simulink model "gm_uz_pmsm_model_9ph"  (R2021b)
settings: Solver=FixedStepAuto  StartTime=0.0  StopTime=0.8  RelTol=1e-3
PreLoadFcn:
  | uz_pmsm_model_9ph_init_parameter
undefined symbols (not defined in the file or in its folder): a, b, c, friction_coefficient, inertia, k_i_d, k_i_q, k_p_d, k_p_q, Kpd, L_d, L_o1, L_o2, L_q, L_x1, L_x2, L_y1, L_y2, L_zero, polepair, psi_pm, R_1, static_friction_torque, Tnd
libraries: hdlmdlgenlib x190, hdlsllib x90, dspsigops x17, simulink x3, slpidlib x2, spsAlphaBetaZerotodq0Lib x1, pid_lib x1, spsdq0toAlphaBetaZeroLib x1
(part 5 of 6)

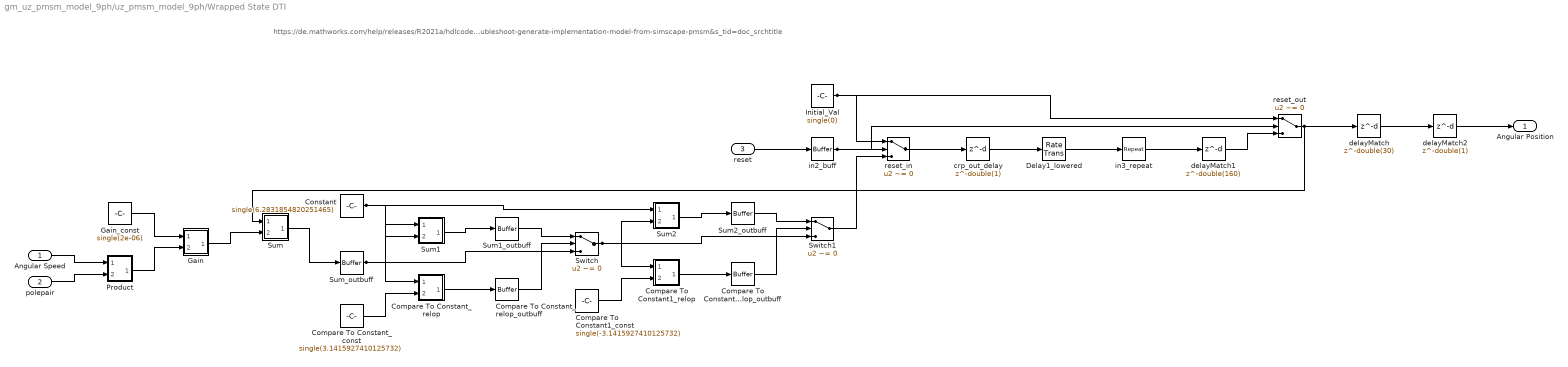
== system gm_uz_pmsm_model_9ph/uz_pmsm_model_9ph/Wrapped State DTI ==
  note: https://de.mathworks.com/help/releases/R2021a/hdlcoder/ug/troubleshoot-generate-implementation-model-from-simscape-pmsm.html?searchHighlight=troubleshoot-generate-implementation-model-from-simscape-pmsm&s_tid=doc_srchtitle
  Angular Speed : Inport  OutDataTypeStr=single  PortDimensions=1  SampleTime=1e-08
  polepair : Inport  Port=2  OutDataTypeStr=single  PortDimensions=1  SampleTime=1e-08
  reset : Inport  Port=3  OutDataTypeStr=boolean  PortDimensions=1  SampleTime=1e-08
  Compare To Constant1_const : Constant  Value=single(-3.1415927410125732)  OutDataTypeStr=single  SampleTime=1e-08
  Compare To Constant1_relop : Subsystem
      mask Display: disp('NFP\nrelop');
  Compare To Constant1_relop_outbuff : hdlmdlgenlib/Buffer
      settings: SourceProductBaseCode=SL
  Compare To Constant_const : Constant  Value=single(3.1415927410125732)  OutDataTypeStr=single  SampleTime=1e-08
  Compare To Constant_relop : Subsystem
      mask Display: disp('NFP\nrelop');
  Compare To Constant_relop_outbuff : hdlmdlgenlib/Buffer
      settings: SourceProductBaseCode=SL
  Constant : Constant  Value=single(6.2831854820251465)  OutDataTypeStr=single  SampleTime=1e-08
  Delay1_lowered : RateTransition  OutPortSampleTimeOpt=Multiple of input port sample time  OutPortSampleTimeMultiple=200
  Gain : Subsystem
      mask Display: disp('NFP\nmul');
  Gain_const : Constant  Value=single(2e-06)  OutDataTypeStr=single  SampleTime=1e-08
  Initial_Val : Constant  Value=single(0)  OutDataTypeStr=single  SampleTime=1e-08
  Product : Subsystem
      mask Display: disp('NFP\nmul');
  Sum : Subsystem
      mask Display: disp('NFP\nadd');
  Sum1 : Subsystem
      mask Display: disp('NFP\nadd');
  Sum1_outbuff : hdlmdlgenlib/Buffer
      settings: SourceProductBaseCode=SL
  Sum2 : Subsystem
      mask Display: disp('NFP\nadd');
  Sum2_outbuff : hdlmdlgenlib/Buffer
      settings: SourceProductBaseCode=SL
  Sum_outbuff : hdlmdlgenlib/Buffer
      settings: SourceProductBaseCode=SL
  Switch : Switch  Criteria=u2 ~= 0  Threshold=double(0)  OutDataTypeStr=single  SampleTime=1e-08
  Switch1 : Switch  Criteria=u2 ~= 0  Threshold=double(0)  OutDataTypeStr=single  SampleTime=1e-08
  crp_out_delay : Delay  DelayLength=double(1)  InitialCondition=0  SampleTime=1e-08
  delayMatch : Delay  DelayLength=double(30)  InitialCondition=0  SampleTime=1e-08
  delayMatch1 : Delay  DelayLength=double(160)  InitialCondition=0  SampleTime=1e-08
  delayMatch2 : Delay  DelayLength=double(1)  InitialCondition=0  SampleTime=1e-08
  in2_buff : hdlmdlgenlib/Buffer
      settings: SourceProductBaseCode=SL
  in3_repeat : dspsigops/Repeat  N=double(200)  RateOptions=Allow multirate processing  ic=0  mode=Unused parameter value
  reset_in : Switch  Criteria=u2 ~= 0  Threshold=double(0)  OutDataTypeStr=single  SampleTime=1e-08
  reset_out : Switch  Criteria=u2 ~= 0  Threshold=double(0)  OutDataTypeStr=single  SampleTime=1e-08
  Angular Position : Outport  SampleTime=1e-08
  wires:
  Angular Speed/1 -> Product/1(In1)
  polepair/1 -> Product/2(In2)
  reset/1 -> in2_buff/1
  Delay1_lowered/1 -> in3_repeat/1
  crp_out_delay/1 -> Delay1_lowered/1
  in3_repeat/1 -> delayMatch1/1
  delayMatch2/1 -> Angular Position/1
  Constant/1 -> Sum2/1(In1), Sum1/2(In2)
  Sum1_outbuff/1 -> Switch/1
  Initial_Val/1 -> reset_out/1, reset_in/1
  Switch1/1 -> reset_in/3
  Sum2_outbuff/1 -> Switch1/1
  reset_in/1 -> crp_out_delay/1
  Compare To Constant1_const/1 -> Compare To Constant1_relop/2(In2)
  Compare To Constant_const/1 -> Compare To Constant_relop/2(In2)
  Gain_const/1 -> Gain/1(In1)
  Sum1/1(Out1) -> Sum1_outbuff/1
  Product/1(Out1) -> Gain/2(In2)
  Sum/1(Out1) -> Sum_outbuff/1
  Compare To Constant1_relop/1(Out1) -> Compare To Constant1_relop_outbuff/1
  Sum2/1(Out1) -> Sum2_outbuff/1
  Compare To Constant_relop/1(Out1) -> Compare To Constant_relop_outbuff/1
  Gain/1(Out1) -> Sum/2(In2)
  in2_buff/1 -> reset_out/2, reset_in/2
  delayMatch1/1 -> reset_out/3
  Compare To Constant_relop_outbuff/1 -> Switch/2
  Sum_outbuff/1 -> Compare To Constant_relop/1(In1), Sum1/1(In1), Switch/3
  Compare To Constant1_relop_outbuff/1 -> Switch1/2
  Switch/1 -> Sum2/2(In2), Compare To Constant1_relop/1(In1), Switch1/3
  reset_out/1 -> delayMatch/1, Sum/1(In1)
  delayMatch/1 -> delayMatch2/1

== system gm_uz_pmsm_model_9ph/uz_pmsm_model_9ph/Line-Line to Phase voltage/Product ==
  In1 : Inport
  In2 : Inport  Port=2
  Product : Product  Inputs=**  OutDataTypeStr=single  SampleTime=1e-08
  Product_pd1 : Delay  DelayLength=6
  Out1 : Outport
  wires:
  In1/1 -> Product/1
  In2/1 -> Product/2
  Product/1 -> Product_pd1/1
  Product_pd1/1 -> Out1/1

== system gm_uz_pmsm_model_9ph/uz_pmsm_model_9ph/Line-Line to Phase voltage/Product1 ==
  In1 : Inport
  In2 : Inport  Port=2
  Product1 : Product  Inputs=**  OutDataTypeStr=single  SampleTime=1e-08
  Product1_pd1 : Delay  DelayLength=6
  Out1 : Outport
  wires:
  In1/1 -> Product1/1
  In2/1 -> Product1/2
  Product1/1 -> Product1_pd1/1
  Product1_pd1/1 -> Out1/1

== system gm_uz_pmsm_model_9ph/uz_pmsm_model_9ph/Line-Line to Phase voltage/Product2 ==
  In1 : Inport
  In2 : Inport  Port=2
  Product2 : Product  Inputs=**  OutDataTypeStr=single  SampleTime=1e-08
  Product2_pd1 : Delay  DelayLength=6
  Out1 : Outport
  wires:
  In1/1 -> Product2/1
  In2/1 -> Product2/2
  Product2/1 -> Product2_pd1/1
  Product2_pd1/1 -> Out1/1

== system gm_uz_pmsm_model_9ph/uz_pmsm_model_9ph/Line-Line to Phase voltage/Product3 ==
  In1 : Inport
  In2 : Inport  Port=2
  Product3 : Product  Inputs=**  OutDataTypeStr=single  SampleTime=1e-08
  Product3_pd1 : Delay  DelayLength=6
  Out1 : Outport
  wires:
  In1/1 -> Product3/1
  In2/1 -> Product3/2
  Product3/1 -> Product3_pd1/1
  Product3_pd1/1 -> Out1/1

== system gm_uz_pmsm_model_9ph/uz_pmsm_model_9ph/Line-Line to Phase voltage/Product_AC_minus_BD ==
  In1 : Inport
  In2 : Inport  Port=2
  Product_AC_minus_BD : Sum  Inputs=+-  OutDataTypeStr=single  SampleTime=1e-08
  Product_AC_minus_BD_pd1 : Delay  DelayLength=6
  Out1 : Outport
  wires:
  In1/1 -> Product_AC_minus_BD/1
  In2/1 -> Product_AC_minus_BD/2
  Product_AC_minus_BD/1 -> Product_AC_minus_BD_pd1/1
  Product_AC_minus_BD_pd1/1 -> Out1/1

== system gm_uz_pmsm_model_9ph/uz_pmsm_model_9ph/Line-Line to Phase voltage/Product_AD_plus_BC ==
  In1 : Inport
  In2 : Inport  Port=2
  Product_AD_plus_BC : Sum  OutDataTypeStr=single  SampleTime=1e-08
  Product_AD_plus_BC_pd1 : Delay  DelayLength=6
  Out1 : Outport
  wires:
  In1/1 -> Product_AD_plus_BC/1
  In2/1 -> Product_AD_plus_BC/2
  Product_AD_plus_BC/1 -> Product_AD_plus_BC_pd1/1
  Product_AD_plus_BC_pd1/1 -> Out1/1

== system gm_uz_pmsm_model_9ph/uz_pmsm_model_9ph/Line-Line to Phase voltage/abc   to   alpha_beta_0 ==
  "a, b, c" : Inport  OutDataTypeStr=single  PortDimensions=[3]  SampleTime=1e-08
  Gain2 : Subsystem
      mask Display: disp('NFP\nmul');
  Gain2_const : Constant  Value=single(0.6666666865348816)  OutDataTypeStr=single  SampleTime=1e-08
  Gain4_const : Constant  Value=single([1 0 0.5 -0.5 0.8660253882408142 0.5 -0.5 -0.8660253882408142 0.5]).'  OutDataTypeStr=single  SampleTime=1e-08
  MMul_add_01 : Subsystem
      mask Display: disp('NFP\nadd');
  MMul_add_12 : Subsystem
      mask Display: disp('NFP\nadd');
  MMul_dot_product : Subsystem
      mask Display: disp('NFP\nmul');
  Reshape : Reshape  OutputDimensionality=Column vector (2-D)
  Row2Col_in0 : Reshape  OutputDimensionality=Column vector (2-D)
  Row2Col_in1 : Reshape  OutputDimensionality=Column vector (2-D)
  delayMatch : Delay  DelayLength=double(6)  InitialCondition=0  SampleTime=1e-08
  delayMatch1 : Delay  DelayLength=double(18)  InitialCondition=0  SampleTime=1e-08
  reshape_dotProduct : Reshape  OutputDimensionality=Customize  OutputDimensions=[3,3]
  reshape_mmulResult : Reshape  OutputDimensionality=Customize  OutputDimensions=[3,1]
  select_0 : Selector  NumberOfDimensions=2  SampleTime=1e-08  IndexOptions=Index vector (dialog),Select all  Indices=double(1),[]  OutputSizes=1
  select_1 : Selector  NumberOfDimensions=2  SampleTime=1e-08  IndexOptions=Index vector (dialog),Select all  Indices=double(2),[]  OutputSizes=1
  select_2 : Selector  NumberOfDimensions=2  SampleTime=1e-08  IndexOptions=Index vector (dialog),Select all  Indices=double(3),[]  OutputSizes=1
  select_indices0 : Selector  SampleTime=1e-08  IndexOptions=Index vector (dialog)  Indices=double([1 4 7 2 5 8 3 6 9])  OutputSizes=1
  select_indices1 : Selector  SampleTime=1e-08  IndexOptions=Index vector (dialog)  Indices=double([1 2 3 1 2 3 1 2 3])  OutputSizes=1
  t : Reshape  OutputDimensionality=Customize  OutputDimensions=[3,3]
  t1 : Mux  Inputs=3
  vectorized_in0 : Reshape  OutputDimensionality=Row vector (2-D)
  "alpha, beta, 0 " : Outport  SampleTime=1e-08
  wires:
  reshape_mmulResult/1 -> Gain2/1(In1)
  Reshape/1 -> select_indices1/1
  t/1 -> vectorized_in0/1
  vectorized_in0/1 -> select_indices0/1
  select_indices0/1 -> Row2Col_in0/1
  select_indices1/1 -> Row2Col_in1/1
  Row2Col_in0/1 -> MMul_dot_product/1(In1)
  Row2Col_in1/1 -> MMul_dot_product/2(In2)
  reshape_dotProduct/1 -> select_2/1, select_1/1, select_0/1
  select_0/1 -> MMul_add_01/1(In1)
  select_1/1 -> MMul_add_01/2(In2)
  delayMatch/1 -> MMul_add_12/2(In2)
  Gain4_const/1 -> t/1
  Gain2_const/1 -> t1/3, t1/2, t1/1
  MMul_dot_product/1(Out1) -> reshape_dotProduct/1
  MMul_add_01/1(Out1) -> MMul_add_12/1(In1)
  MMul_add_12/1(Out1) -> reshape_mmulResult/1
  delayMatch1/1 -> Gain2/2(In2)
  Gain2/1(Out1) -> "alpha, beta, 0 "/1
  select_2/1 -> delayMatch/1
  t1/1 -> delayMatch1/1
  "a, b, c"/1 -> Reshape/1

== system gm_uz_pmsm_model_9ph/uz_pmsm_model_9ph/Line-Line to Phase voltage/alpha_beta_0   to   abc ==
  "alpha, beta, 0  " : Inport  OutDataTypeStr=single  PortDimensions=[3]  SampleTime=1e-08
  Gain4_const : Constant  Value=single([1 -0.5 -0.5 0 0.8660253882408142 -0.8660253882408142 1 1 1]).'  OutDataTypeStr=single  SampleTime=1e-08
  MMul_add_01 : Subsystem
      mask Display: disp('NFP\nadd');
  MMul_add_12 : Subsystem
      mask Display: disp('NFP\nadd');
  MMul_dot_product : Subsystem
      mask Display: disp('NFP\nmul');
  Reshape : Reshape  OutputDimensionality=Column vector (2-D)
  Row2Col_in0 : Reshape  OutputDimensionality=Column vector (2-D)
  Row2Col_in1 : Reshape  OutputDimensionality=Column vector (2-D)
  delayMatch : Delay  DelayLength=double(6)  InitialCondition=0  SampleTime=1e-08
  reshape_dotProduct : Reshape  OutputDimensionality=Customize  OutputDimensions=[3,3]
  reshape_mmulResult : Reshape  OutputDimensionality=Customize  OutputDimensions=[3,1]
  select_0 : Selector  NumberOfDimensions=2  SampleTime=1e-08  IndexOptions=Index vector (dialog),Select all  Indices=double(1),[]  OutputSizes=1
  select_1 : Selector  NumberOfDimensions=2  SampleTime=1e-08  IndexOptions=Index vector (dialog),Select all  Indices=double(2),[]  OutputSizes=1
  select_2 : Selector  NumberOfDimensions=2  SampleTime=1e-08  IndexOptions=Index vector (dialog),Select all  Indices=double(3),[]  OutputSizes=1
  select_indices0 : Selector  SampleTime=1e-08  IndexOptions=Index vector (dialog)  Indices=double([1 4 7 2 5 8 3 6 9])  OutputSizes=1
  select_indices1 : Selector  SampleTime=1e-08  IndexOptions=Index vector (dialog)  Indices=double([1 2 3 1 2 3 1 2 3])  OutputSizes=1
  t : Reshape  OutputDimensionality=Customize  OutputDimensions=[3,3]
  vectorized_in0 : Reshape  OutputDimensionality=Row vector (2-D)
  "a, b, c" : Outport  SampleTime=1e-08
  wires:
  reshape_mmulResult/1 -> "a, b, c"/1
  Reshape/1 -> select_indices1/1
  t/1 -> vectorized_in0/1
  vectorized_in0/1 -> select_indices0/1
  select_indices0/1 -> Row2Col_in0/1
  select_indices1/1 -> Row2Col_in1/1
  Row2Col_in0/1 -> MMul_dot_product/1(In1)
  Row2Col_in1/1 -> MMul_dot_product/2(In2)
  reshape_dotProduct/1 -> select_2/1, select_1/1, select_0/1
  select_0/1 -> MMul_add_01/1(In1)
  select_1/1 -> MMul_add_01/2(In2)
  delayMatch/1 -> MMul_add_12/2(In2)
  Gain4_const/1 -> t/1
  MMul_dot_product/1(Out1) -> reshape_dotProduct/1
  MMul_add_01/1(Out1) -> MMul_add_12/1(In1)
  MMul_add_12/1(Out1) -> reshape_mmulResult/1
  select_2/1 -> delayMatch/1
  "alpha, beta, 0  "/1 -> Reshape/1

== system gm_uz_pmsm_model_9ph/uz_pmsm_model_9ph/Line-Line to Phase voltage1/Product ==
  In1 : Inport
  In2 : Inport  Port=2
  Product : Product  Inputs=**  OutDataTypeStr=single  SampleTime=1e-08
  Product_pd1 : Delay  DelayLength=6
  Out1 : Outport
  wires:
  In1/1 -> Product/1
  In2/1 -> Product/2
  Product/1 -> Product_pd1/1
  Product_pd1/1 -> Out1/1

== system gm_uz_pmsm_model_9ph/uz_pmsm_model_9ph/Line-Line to Phase voltage1/Product1 ==
  In1 : Inport
  In2 : Inport  Port=2
  Product1 : Product  Inputs=**  OutDataTypeStr=single  SampleTime=1e-08
  Product1_pd1 : Delay  DelayLength=6
  Out1 : Outport
  wires:
  In1/1 -> Product1/1
  In2/1 -> Product1/2
  Product1/1 -> Product1_pd1/1
  Product1_pd1/1 -> Out1/1

== system gm_uz_pmsm_model_9ph/uz_pmsm_model_9ph/Line-Line to Phase voltage1/Product2 ==
  In1 : Inport
  In2 : Inport  Port=2
  Product2 : Product  Inputs=**  OutDataTypeStr=single  SampleTime=1e-08
  Product2_pd1 : Delay  DelayLength=6
  Out1 : Outport
  wires:
  In1/1 -> Product2/1
  In2/1 -> Product2/2
  Product2/1 -> Product2_pd1/1
  Product2_pd1/1 -> Out1/1

== system gm_uz_pmsm_model_9ph/uz_pmsm_model_9ph/Line-Line to Phase voltage1/Product3 ==
  In1 : Inport
  In2 : Inport  Port=2
  Product3 : Product  Inputs=**  OutDataTypeStr=single  SampleTime=1e-08
  Product3_pd1 : Delay  DelayLength=6
  Out1 : Outport
  wires:
  In1/1 -> Product3/1
  In2/1 -> Product3/2
  Product3/1 -> Product3_pd1/1
  Product3_pd1/1 -> Out1/1

== system gm_uz_pmsm_model_9ph/uz_pmsm_model_9ph/Line-Line to Phase voltage1/Product_AC_minus_BD ==
  In1 : Inport
  In2 : Inport  Port=2
  Product_AC_minus_BD : Sum  Inputs=+-  OutDataTypeStr=single  SampleTime=1e-08
  Product_AC_minus_BD_pd1 : Delay  DelayLength=6
  Out1 : Outport
  wires:
  In1/1 -> Product_AC_minus_BD/1
  In2/1 -> Product_AC_minus_BD/2
  Product_AC_minus_BD/1 -> Product_AC_minus_BD_pd1/1
  Product_AC_minus_BD_pd1/1 -> Out1/1

== system gm_uz_pmsm_model_9ph/uz_pmsm_model_9ph/Line-Line to Phase voltage1/Product_AD_plus_BC ==
  In1 : Inport
  In2 : Inport  Port=2
  Product_AD_plus_BC : Sum  OutDataTypeStr=single  SampleTime=1e-08
  Product_AD_plus_BC_pd1 : Delay  DelayLength=6
  Out1 : Outport
  wires:
  In1/1 -> Product_AD_plus_BC/1
  In2/1 -> Product_AD_plus_BC/2
  Product_AD_plus_BC/1 -> Product_AD_plus_BC_pd1/1
  Product_AD_plus_BC_pd1/1 -> Out1/1

== system gm_uz_pmsm_model_9ph/uz_pmsm_model_9ph/Line-Line to Phase voltage1/abc   to   alpha_beta_0 ==
  "a, b, c" : Inport  OutDataTypeStr=single  PortDimensions=[3]  SampleTime=1e-08
  Gain2 : Subsystem
      mask Display: disp('NFP\nmul');
  Gain2_const : Constant  Value=single(0.6666666865348816)  OutDataTypeStr=single  SampleTime=1e-08
  Gain4_const : Constant  Value=single([1 0 0.5 -0.5 0.8660253882408142 0.5 -0.5 -0.8660253882408142 0.5]).'  OutDataTypeStr=single  SampleTime=1e-08
  MMul_add_01 : Subsystem
      mask Display: disp('NFP\nadd');
  MMul_add_12 : Subsystem
      mask Display: disp('NFP\nadd');
  MMul_dot_product : Subsystem
      mask Display: disp('NFP\nmul');
  Reshape : Reshape  OutputDimensionality=Column vector (2-D)
  Row2Col_in0 : Reshape  OutputDimensionality=Column vector (2-D)
  Row2Col_in1 : Reshape  OutputDimensionality=Column vector (2-D)
  delayMatch : Delay  DelayLength=double(6)  InitialCondition=0  SampleTime=1e-08
  delayMatch1 : Delay  DelayLength=double(18)  InitialCondition=0  SampleTime=1e-08
  reshape_dotProduct : Reshape  OutputDimensionality=Customize  OutputDimensions=[3,3]
  reshape_mmulResult : Reshape  OutputDimensionality=Customize  OutputDimensions=[3,1]
  select_0 : Selector  NumberOfDimensions=2  SampleTime=1e-08  IndexOptions=Index vector (dialog),Select all  Indices=double(1),[]  OutputSizes=1
  select_1 : Selector  NumberOfDimensions=2  SampleTime=1e-08  IndexOptions=Index vector (dialog),Select all  Indices=double(2),[]  OutputSizes=1
  select_2 : Selector  NumberOfDimensions=2  SampleTime=1e-08  IndexOptions=Index vector (dialog),Select all  Indices=double(3),[]  OutputSizes=1
  select_indices0 : Selector  SampleTime=1e-08  IndexOptions=Index vector (dialog)  Indices=double([1 4 7 2 5 8 3 6 9])  OutputSizes=1
  select_indices1 : Selector  SampleTime=1e-08  IndexOptions=Index vector (dialog)  Indices=double([1 2 3 1 2 3 1 2 3])  OutputSizes=1
  t : Reshape  OutputDimensionality=Customize  OutputDimensions=[3,3]
  t1 : Mux  Inputs=3
  vectorized_in0 : Reshape  OutputDimensionality=Row vector (2-D)
  "alpha, beta, 0 " : Outport  SampleTime=1e-08
  wires:
  reshape_mmulResult/1 -> Gain2/1(In1)
  Reshape/1 -> select_indices1/1
  t/1 -> vectorized_in0/1
  vectorized_in0/1 -> select_indices0/1
  select_indices0/1 -> Row2Col_in0/1
  select_indices1/1 -> Row2Col_in1/1
  Row2Col_in0/1 -> MMul_dot_product/1(In1)
  Row2Col_in1/1 -> MMul_dot_product/2(In2)
  reshape_dotProduct/1 -> select_2/1, select_1/1, select_0/1
  select_0/1 -> MMul_add_01/1(In1)
  select_1/1 -> MMul_add_01/2(In2)
  delayMatch/1 -> MMul_add_12/2(In2)
  Gain4_const/1 -> t/1
  Gain2_const/1 -> t1/3, t1/2, t1/1
  MMul_dot_product/1(Out1) -> reshape_dotProduct/1
  MMul_add_01/1(Out1) -> MMul_add_12/1(In1)
  MMul_add_12/1(Out1) -> reshape_mmulResult/1
  delayMatch1/1 -> Gain2/2(In2)
  Gain2/1(Out1) -> "alpha, beta, 0 "/1
  select_2/1 -> delayMatch/1
  t1/1 -> delayMatch1/1
  "a, b, c"/1 -> Reshape/1

== system gm_uz_pmsm_model_9ph/uz_pmsm_model_9ph/Line-Line to Phase voltage1/alpha_beta_0   to   abc ==
  "alpha, beta, 0  " : Inport  OutDataTypeStr=single  PortDimensions=[3]  SampleTime=1e-08
  Gain4_const : Constant  Value=single([1 -0.5 -0.5 0 0.8660253882408142 -0.8660253882408142 1 1 1]).'  OutDataTypeStr=single  SampleTime=1e-08
  MMul_add_01 : Subsystem
      mask Display: disp('NFP\nadd');
  MMul_add_12 : Subsystem
      mask Display: disp('NFP\nadd');
  MMul_dot_product : Subsystem
      mask Display: disp('NFP\nmul');
  Reshape : Reshape  OutputDimensionality=Column vector (2-D)
  Row2Col_in0 : Reshape  OutputDimensionality=Column vector (2-D)
  Row2Col_in1 : Reshape  OutputDimensionality=Column vector (2-D)
  delayMatch : Delay  DelayLength=double(6)  InitialCondition=0  SampleTime=1e-08
  reshape_dotProduct : Reshape  OutputDimensionality=Customize  OutputDimensions=[3,3]
  reshape_mmulResult : Reshape  OutputDimensionality=Customize  OutputDimensions=[3,1]
  select_0 : Selector  NumberOfDimensions=2  SampleTime=1e-08  IndexOptions=Index vector (dialog),Select all  Indices=double(1),[]  OutputSizes=1
  select_1 : Selector  NumberOfDimensions=2  SampleTime=1e-08  IndexOptions=Index vector (dialog),Select all  Indices=double(2),[]  OutputSizes=1
  select_2 : Selector  NumberOfDimensions=2  SampleTime=1e-08  IndexOptions=Index vector (dialog),Select all  Indices=double(3),[]  OutputSizes=1
  select_indices0 : Selector  SampleTime=1e-08  IndexOptions=Index vector (dialog)  Indices=double([1 4 7 2 5 8 3 6 9])  OutputSizes=1
  select_indices1 : Selector  SampleTime=1e-08  IndexOptions=Index vector (dialog)  Indices=double([1 2 3 1 2 3 1 2 3])  OutputSizes=1
  t : Reshape  OutputDimensionality=Customize  OutputDimensions=[3,3]
  vectorized_in0 : Reshape  OutputDimensionality=Row vector (2-D)
  "a, b, c" : Outport  SampleTime=1e-08
  wires:
  reshape_mmulResult/1 -> "a, b, c"/1
  Reshape/1 -> select_indices1/1
  t/1 -> vectorized_in0/1
  vectorized_in0/1 -> select_indices0/1
  select_indices0/1 -> Row2Col_in0/1
  select_indices1/1 -> Row2Col_in1/1
  Row2Col_in0/1 -> MMul_dot_product/1(In1)
  Row2Col_in1/1 -> MMul_dot_product/2(In2)
  reshape_dotProduct/1 -> select_2/1, select_1/1, select_0/1
  select_0/1 -> MMul_add_01/1(In1)
  select_1/1 -> MMul_add_01/2(In2)
  delayMatch/1 -> MMul_add_12/2(In2)
  Gain4_const/1 -> t/1
  MMul_dot_product/1(Out1) -> reshape_dotProduct/1
  MMul_add_01/1(Out1) -> MMul_add_12/1(In1)
  MMul_add_12/1(Out1) -> reshape_mmulResult/1
  select_2/1 -> delayMatch/1
  "alpha, beta, 0  "/1 -> Reshape/1

== system gm_uz_pmsm_model_9ph/uz_pmsm_model_9ph/Line-Line to Phase voltage2/Product ==
  In1 : Inport
  In2 : Inport  Port=2
  Product : Product  Inputs=**  OutDataTypeStr=single  SampleTime=1e-08
  Product_pd1 : Delay  DelayLength=6
  Out1 : Outport
  wires:
  In1/1 -> Product/1
  In2/1 -> Product/2
  Product/1 -> Product_pd1/1
  Product_pd1/1 -> Out1/1

== system gm_uz_pmsm_model_9ph/uz_pmsm_model_9ph/Line-Line to Phase voltage2/Product1 ==
  In1 : Inport
  In2 : Inport  Port=2
  Product1 : Product  Inputs=**  OutDataTypeStr=single  SampleTime=1e-08
  Product1_pd1 : Delay  DelayLength=6
  Out1 : Outport
  wires:
  In1/1 -> Product1/1
  In2/1 -> Product1/2
  Product1/1 -> Product1_pd1/1
  Product1_pd1/1 -> Out1/1

== system gm_uz_pmsm_model_9ph/uz_pmsm_model_9ph/Line-Line to Phase voltage2/Product2 ==
  In1 : Inport
  In2 : Inport  Port=2
  Product2 : Product  Inputs=**  OutDataTypeStr=single  SampleTime=1e-08
  Product2_pd1 : Delay  DelayLength=6
  Out1 : Outport
  wires:
  In1/1 -> Product2/1
  In2/1 -> Product2/2
  Product2/1 -> Product2_pd1/1
  Product2_pd1/1 -> Out1/1

== system gm_uz_pmsm_model_9ph/uz_pmsm_model_9ph/Line-Line to Phase voltage2/Product3 ==
  In1 : Inport
  In2 : Inport  Port=2
  Product3 : Product  Inputs=**  OutDataTypeStr=single  SampleTime=1e-08
  Product3_pd1 : Delay  DelayLength=6
  Out1 : Outport
  wires:
  In1/1 -> Product3/1
  In2/1 -> Product3/2
  Product3/1 -> Product3_pd1/1
  Product3_pd1/1 -> Out1/1

== system gm_uz_pmsm_model_9ph/uz_pmsm_model_9ph/Line-Line to Phase voltage2/Product_AC_minus_BD ==
  In1 : Inport
  In2 : Inport  Port=2
  Product_AC_minus_BD : Sum  Inputs=+-  OutDataTypeStr=single  SampleTime=1e-08
  Product_AC_minus_BD_pd1 : Delay  DelayLength=6
  Out1 : Outport
  wires:
  In1/1 -> Product_AC_minus_BD/1
  In2/1 -> Product_AC_minus_BD/2
  Product_AC_minus_BD/1 -> Product_AC_minus_BD_pd1/1
  Product_AC_minus_BD_pd1/1 -> Out1/1

== system gm_uz_pmsm_model_9ph/uz_pmsm_model_9ph/Line-Line to Phase voltage2/Product_AD_plus_BC ==
  In1 : Inport
  In2 : Inport  Port=2
  Product_AD_plus_BC : Sum  OutDataTypeStr=single  SampleTime=1e-08
  Product_AD_plus_BC_pd1 : Delay  DelayLength=6
  Out1 : Outport
  wires:
  In1/1 -> Product_AD_plus_BC/1
  In2/1 -> Product_AD_plus_BC/2
  Product_AD_plus_BC/1 -> Product_AD_plus_BC_pd1/1
  Product_AD_plus_BC_pd1/1 -> Out1/1

== system gm_uz_pmsm_model_9ph/uz_pmsm_model_9ph/Line-Line to Phase voltage2/abc   to   alpha_beta_0 ==
  "a, b, c" : Inport  OutDataTypeStr=single  PortDimensions=[3]  SampleTime=1e-08
  Gain2 : Subsystem
      mask Display: disp('NFP\nmul');
  Gain2_const : Constant  Value=single(0.6666666865348816)  OutDataTypeStr=single  SampleTime=1e-08
  Gain4_const : Constant  Value=single([1 0 0.5 -0.5 0.8660253882408142 0.5 -0.5 -0.8660253882408142 0.5]).'  OutDataTypeStr=single  SampleTime=1e-08
  MMul_add_01 : Subsystem
      mask Display: disp('NFP\nadd');
  MMul_add_12 : Subsystem
      mask Display: disp('NFP\nadd');
  MMul_dot_product : Subsystem
      mask Display: disp('NFP\nmul');
  Reshape : Reshape  OutputDimensionality=Column vector (2-D)
  Row2Col_in0 : Reshape  OutputDimensionality=Column vector (2-D)
  Row2Col_in1 : Reshape  OutputDimensionality=Column vector (2-D)
  delayMatch : Delay  DelayLength=double(6)  InitialCondition=0  SampleTime=1e-08
  delayMatch1 : Delay  DelayLength=double(18)  InitialCondition=0  SampleTime=1e-08
  reshape_dotProduct : Reshape  OutputDimensionality=Customize  OutputDimensions=[3,3]
  reshape_mmulResult : Reshape  OutputDimensionality=Customize  OutputDimensions=[3,1]
  select_0 : Selector  NumberOfDimensions=2  SampleTime=1e-08  IndexOptions=Index vector (dialog),Select all  Indices=double(1),[]  OutputSizes=1
  select_1 : Selector  NumberOfDimensions=2  SampleTime=1e-08  IndexOptions=Index vector (dialog),Select all  Indices=double(2),[]  OutputSizes=1
  select_2 : Selector  NumberOfDimensions=2  SampleTime=1e-08  IndexOptions=Index vector (dialog),Select all  Indices=double(3),[]  OutputSizes=1
  select_indices0 : Selector  SampleTime=1e-08  IndexOptions=Index vector (dialog)  Indices=double([1 4 7 2 5 8 3 6 9])  OutputSizes=1
  select_indices1 : Selector  SampleTime=1e-08  IndexOptions=Index vector (dialog)  Indices=double([1 2 3 1 2 3 1 2 3])  OutputSizes=1
  t : Reshape  OutputDimensionality=Customize  OutputDimensions=[3,3]
  t1 : Mux  Inputs=3
  vectorized_in0 : Reshape  OutputDimensionality=Row vector (2-D)
  "alpha, beta, 0 " : Outport  SampleTime=1e-08
  wires:
  reshape_mmulResult/1 -> Gain2/1(In1)
  Reshape/1 -> select_indices1/1
  t/1 -> vectorized_in0/1
  vectorized_in0/1 -> select_indices0/1
  select_indices0/1 -> Row2Col_in0/1
  select_indices1/1 -> Row2Col_in1/1
  Row2Col_in0/1 -> MMul_dot_product/1(In1)
  Row2Col_in1/1 -> MMul_dot_product/2(In2)
  reshape_dotProduct/1 -> select_2/1, select_1/1, select_0/1
  select_0/1 -> MMul_add_01/1(In1)
  select_1/1 -> MMul_add_01/2(In2)
  delayMatch/1 -> MMul_add_12/2(In2)
  Gain4_const/1 -> t/1
  Gain2_const/1 -> t1/3, t1/2, t1/1
  MMul_dot_product/1(Out1) -> reshape_dotProduct/1
  MMul_add_01/1(Out1) -> MMul_add_12/1(In1)
  MMul_add_12/1(Out1) -> reshape_mmulResult/1
  delayMatch1/1 -> Gain2/2(In2)
  Gain2/1(Out1) -> "alpha, beta, 0 "/1
  select_2/1 -> delayMatch/1
  t1/1 -> delayMatch1/1
  "a, b, c"/1 -> Reshape/1

== system gm_uz_pmsm_model_9ph/uz_pmsm_model_9ph/Line-Line to Phase voltage2/alpha_beta_0   to   abc ==
  "alpha, beta, 0  " : Inport  OutDataTypeStr=single  PortDimensions=[3]  SampleTime=1e-08
  Gain4_const : Constant  Value=single([1 -0.5 -0.5 0 0.8660253882408142 -0.8660253882408142 1 1 1]).'  OutDataTypeStr=single  SampleTime=1e-08
  MMul_add_01 : Subsystem
      mask Display: disp('NFP\nadd');
  MMul_add_12 : Subsystem
      mask Display: disp('NFP\nadd');
  MMul_dot_product : Subsystem
      mask Display: disp('NFP\nmul');
  Reshape : Reshape  OutputDimensionality=Column vector (2-D)
  Row2Col_in0 : Reshape  OutputDimensionality=Column vector (2-D)
  Row2Col_in1 : Reshape  OutputDimensionality=Column vector (2-D)
  delayMatch : Delay  DelayLength=double(6)  InitialCondition=0  SampleTime=1e-08
  reshape_dotProduct : Reshape  OutputDimensionality=Customize  OutputDimensions=[3,3]
  reshape_mmulResult : Reshape  OutputDimensionality=Customize  OutputDimensions=[3,1]
  select_0 : Selector  NumberOfDimensions=2  SampleTime=1e-08  IndexOptions=Index vector (dialog),Select all  Indices=double(1),[]  OutputSizes=1
  select_1 : Selector  NumberOfDimensions=2  SampleTime=1e-08  IndexOptions=Index vector (dialog),Select all  Indices=double(2),[]  OutputSizes=1
  select_2 : Selector  NumberOfDimensions=2  SampleTime=1e-08  IndexOptions=Index vector (dialog),Select all  Indices=double(3),[]  OutputSizes=1
  select_indices0 : Selector  SampleTime=1e-08  IndexOptions=Index vector (dialog)  Indices=double([1 4 7 2 5 8 3 6 9])  OutputSizes=1
  select_indices1 : Selector  SampleTime=1e-08  IndexOptions=Index vector (dialog)  Indices=double([1 2 3 1 2 3 1 2 3])  OutputSizes=1
  t : Reshape  OutputDimensionality=Customize  OutputDimensions=[3,3]
  vectorized_in0 : Reshape  OutputDimensionality=Row vector (2-D)
  "a, b, c" : Outport  SampleTime=1e-08
  wires:
  reshape_mmulResult/1 -> "a, b, c"/1
  Reshape/1 -> select_indices1/1
  t/1 -> vectorized_in0/1
  vectorized_in0/1 -> select_indices0/1
  select_indices0/1 -> Row2Col_in0/1
  select_indices1/1 -> Row2Col_in1/1
  Row2Col_in0/1 -> MMul_dot_product/1(In1)
  Row2Col_in1/1 -> MMul_dot_product/2(In2)
  reshape_dotProduct/1 -> select_2/1, select_1/1, select_0/1
  select_0/1 -> MMul_add_01/1(In1)
  select_1/1 -> MMul_add_01/2(In2)
  delayMatch/1 -> MMul_add_12/2(In2)
  Gain4_const/1 -> t/1
  MMul_dot_product/1(Out1) -> reshape_dotProduct/1
  MMul_add_01/1(Out1) -> MMul_add_12/1(In1)
  MMul_add_12/1(Out1) -> reshape_mmulResult/1
  select_2/1 -> delayMatch/1
  "alpha, beta, 0  "/1 -> Reshape/1

== system gm_uz_pmsm_model_9ph/uz_pmsm_model_9ph/Transformation/Add ==
  In1 : Inport
  In2 : Inport  Port=2
  Add : Sum  OutDataTypeStr=single  SampleTime=1e-08
  Add_pd1 : Delay  DelayLength=6
  Out1 : Outport
  wires:
  In1/1 -> Add/1
  In2/1 -> Add/2
  Add/1 -> Add_pd1/1
  Add_pd1/1 -> Out1/1

== system gm_uz_pmsm_model_9ph/uz_pmsm_model_9ph/Transformation/Add1 ==
  In1 : Inport
  In2 : Inport  Port=2
  Add1 : Sum  Inputs=+-  OutDataTypeStr=single  SampleTime=1e-08
  Add1_pd1 : Delay  DelayLength=6
  Out1 : Outport
  wires:
  In1/1 -> Add1/1
  In2/1 -> Add1/2
  Add1/1 -> Add1_pd1/1
  Add1_pd1/1 -> Out1/1

== system gm_uz_pmsm_model_9ph/uz_pmsm_model_9ph/Transformation/Data Type Conversion39 ==
  In1 : Inport
  Data Type Conversion39 : DataTypeConversion  OutDataTypeStr=single  RndMeth=Nearest  SampleTime=1e-08
  Data Type Conversion39_pd1 : Delay  DelayLength=6
  Out1 : Outport
  wires:
  In1/1 -> Data Type Conversion39/1
  Data Type Conversion39/1 -> Data Type Conversion39_pd1/1
  Data Type Conversion39_pd1/1 -> Out1/1

== system gm_uz_pmsm_model_9ph/uz_pmsm_model_9ph/Transformation/Divide ==
  In1 : Inport
  In2 : Inport  Port=2
  Divide : Product  Inputs=**  OutDataTypeStr=single  SampleTime=1e-08
  Divide_pd1 : Delay  DelayLength=6
  Out1 : Outport
  wires:
  In1/1 -> Divide/1
  In2/1 -> Divide/2
  Divide/1 -> Divide_pd1/1
  Divide_pd1/1 -> Out1/1

== system gm_uz_pmsm_model_9ph/uz_pmsm_model_9ph/Transformation/Divide1 ==
  In1 : Inport
  In2 : Inport  Port=2
  Divide1 : Product  Inputs=**  OutDataTypeStr=single  SampleTime=1e-08
  Divide1_pd1 : Delay  DelayLength=6
  Out1 : Outport
  wires:
  In1/1 -> Divide1/1
  In2/1 -> Divide1/2
  Divide1/1 -> Divide1_pd1/1
  Divide1_pd1/1 -> Out1/1

== system gm_uz_pmsm_model_9ph/uz_pmsm_model_9ph/Transformation/Divide2 ==
  In1 : Inport
  In2 : Inport  Port=2
  Divide2 : Product  Inputs=**  OutDataTypeStr=single  SampleTime=1e-08
  Divide2_pd1 : Delay  DelayLength=6
  Out1 : Outport
  wires:
  In1/1 -> Divide2/1
  In2/1 -> Divide2/2
  Divide2/1 -> Divide2_pd1/1
  Divide2_pd1/1 -> Out1/1

== system gm_uz_pmsm_model_9ph/uz_pmsm_model_9ph/Transformation/Divide3 ==
  In1 : Inport
  In2 : Inport  Port=2
  Divide3 : Product  Inputs=**  OutDataTypeStr=single  SampleTime=1e-08
  Divide3_pd1 : Delay  DelayLength=6
  Out1 : Outport
  wires:
  In1/1 -> Divide3/1
  In2/1 -> Divide3/2
  Divide3/1 -> Divide3_pd1/1
  Divide3_pd1/1 -> Out1/1

== system gm_uz_pmsm_model_9ph/uz_pmsm_model_9ph/Transformation/t3 ==
  in0 : Inport
  ColVec1 : Selector  NumberOfDimensions=2  IndexOptions=Select all,Index vector (dialog)  Indices=1,1  OutputSizes=1,1
  ColVec2 : Selector  NumberOfDimensions=2  IndexOptions=Select all,Index vector (dialog)  Indices=1,2  OutputSizes=1,1
  ColVec3 : Selector  NumberOfDimensions=2  IndexOptions=Select all,Index vector (dialog)  Indices=1,3  OutputSizes=1,1
  ColVec4 : Selector  NumberOfDimensions=2  IndexOptions=Select all,Index vector (dialog)  Indices=1,4  OutputSizes=1,1
  ColVec5 : Selector  NumberOfDimensions=2  IndexOptions=Select all,Index vector (dialog)  Indices=1,5  OutputSizes=1,1
  ColVec6 : Selector  NumberOfDimensions=2  IndexOptions=Select all,Index vector (dialog)  Indices=1,6  OutputSizes=1,1
  ColVec7 : Selector  NumberOfDimensions=2  IndexOptions=Select all,Index vector (dialog)  Indices=1,7  OutputSizes=1,1
  ColVec8 : Selector  NumberOfDimensions=2  IndexOptions=Select all,Index vector (dialog)  Indices=1,8  OutputSizes=1,1
  ColVec9 : Selector  NumberOfDimensions=2  IndexOptions=Select all,Index vector (dialog)  Indices=1,9  OutputSizes=1,1
  out0 : Outport
  out1 : Outport  Port=2
  out2 : Outport  Port=3
  out3 : Outport  Port=4
  out4 : Outport  Port=5
  out5 : Outport  Port=6
  out6 : Outport  Port=7
  out7 : Outport  Port=8
  out8 : Outport  Port=9
  wires:
  in0/1 -> ColVec1/1, ColVec2/1, ColVec3/1, ColVec4/1, ColVec5/1, ColVec6/1, ColVec7/1, ColVec8/1, ColVec9/1
  ColVec1/1 -> out0/1
  ColVec2/1 -> out1/1
  ColVec3/1 -> out2/1
  ColVec4/1 -> out3/1
  ColVec5/1 -> out4/1
  ColVec6/1 -> out5/1
  ColVec7/1 -> out6/1
  ColVec8/1 -> out7/1
  ColVec9/1 -> out8/1

== system gm_uz_pmsm_model_9ph/uz_pmsm_model_9ph/Transformation1/Add ==
  In1 : Inport
  In2 : Inport  Port=2
  Add : Sum  Inputs=+-  OutDataTypeStr=single  SampleTime=1e-08
  Add_pd1 : Delay  DelayLength=6
  Out1 : Outport
  wires:
  In1/1 -> Add/1
  In2/1 -> Add/2
  Add/1 -> Add_pd1/1
  Add_pd1/1 -> Out1/1

== system gm_uz_pmsm_model_9ph/uz_pmsm_model_9ph/Transformation1/Add1 ==
  In1 : Inport
  In2 : Inport  Port=2
  Add1 : Sum  OutDataTypeStr=single  SampleTime=1e-08
  Add1_pd1 : Delay  DelayLength=6
  Out1 : Outport
  wires:
  In1/1 -> Add1/1
  In2/1 -> Add1/2
  Add1/1 -> Add1_pd1/1
  Add1_pd1/1 -> Out1/1

== system gm_uz_pmsm_model_9ph/uz_pmsm_model_9ph/Transformation1/Data Type Conversion28 ==
  In1 : Inport
  Data Type Conversion28 : DataTypeConversion  OutDataTypeStr=fixdt(1, 25, 12)  RndMeth=Nearest  SampleTime=1e-08
  Data Type Conversion28_pd1 : Delay  DelayLength=6
  Out1 : Outport
  wires:
  In1/1 -> Data Type Conversion28/1
  Data Type Conversion28/1 -> Data Type Conversion28_pd1/1
  Data Type Conversion28_pd1/1 -> Out1/1

== system gm_uz_pmsm_model_9ph/uz_pmsm_model_9ph/Transformation1/Divide ==
  In1 : Inport
  In2 : Inport  Port=2
  Divide : Product  Inputs=**  OutDataTypeStr=single  SampleTime=1e-08
  Divide_pd1 : Delay  DelayLength=6
  Out1 : Outport
  wires:
  In1/1 -> Divide/1
  In2/1 -> Divide/2
  Divide/1 -> Divide_pd1/1
  Divide_pd1/1 -> Out1/1

== system gm_uz_pmsm_model_9ph/uz_pmsm_model_9ph/Transformation1/Divide1 ==
  In1 : Inport
  In2 : Inport  Port=2
  Divide1 : Product  Inputs=**  OutDataTypeStr=single  SampleTime=1e-08
  Divide1_pd1 : Delay  DelayLength=6
  Out1 : Outport
  wires:
  In1/1 -> Divide1/1
  In2/1 -> Divide1/2
  Divide1/1 -> Divide1_pd1/1
  Divide1_pd1/1 -> Out1/1

== system gm_uz_pmsm_model_9ph/uz_pmsm_model_9ph/Transformation1/Divide2 ==
  In1 : Inport
  In2 : Inport  Port=2
  Divide2 : Product  Inputs=**  OutDataTypeStr=single  SampleTime=1e-08
  Divide2_pd1 : Delay  DelayLength=6
  Out1 : Outport
  wires:
  In1/1 -> Divide2/1
  In2/1 -> Divide2/2
  Divide2/1 -> Divide2_pd1/1
  Divide2_pd1/1 -> Out1/1

== system gm_uz_pmsm_model_9ph/uz_pmsm_model_9ph/Transformation1/Divide3 ==
  In1 : Inport
  In2 : Inport  Port=2
  Divide3 : Product  Inputs=**  OutDataTypeStr=single  SampleTime=1e-08
  Divide3_pd1 : Delay  DelayLength=6
  Out1 : Outport
  wires:
  In1/1 -> Divide3/1
  In2/1 -> Divide3/2
  Divide3/1 -> Divide3_pd1/1
  Divide3_pd1/1 -> Out1/1

== system gm_uz_pmsm_model_9ph/uz_pmsm_model_9ph/Transformation1/Transformation1_MAC ==
  in0 : Inport  OutDataTypeStr=fixdt(1, 18, 16)  PortDimensions=[9 1]  SampleTime=1e-08
  in1 : Inport  Port=2  OutDataTypeStr=fixdt(1, 25, 12)  PortDimensions=[9]  SampleTime=1e-08
  globalSchedule : EnablePort  OutDataTypeStr=boolean
  PipelineRegister : Delay  DelayLength=double(8)  InitialCondition=0
  t : hdlsllib/HDL Operations/Multiply-Accumulate  opMode=Vector  initValueSetting=Dialog  initValue=0  initValueSetting2=Dialog  initValue2=0  initValueSetting3=Dialog  initValue3=0  num_samples=2  RndMeth2=Floor  RndMeth3=Floor  OutDataTypeStr=fixdt(1, 43, 28)  datatype2=Inherit: Inherit via back propagation  datatype3=Inherit: Inherit via back propagation  validOut=on  endInandOut=on  startOut=on  countOut=on  dim=-1  DoSatur=off  parallel=off
      settings: SourceProductBaseCode=SL
  out0 : Outport  OutDataTypeStr=fixdt(1, 43, 28)  SampleTime=1e-08  InitialOutput=0
  wires:
  PipelineRegister/1 -> out0/1
  in0/1 -> t/1
  in1/1 -> t/2
  t/1 -> PipelineRegister/1

== system gm_uz_pmsm_model_9ph/uz_pmsm_model_9ph/Transformation1/Transformation1_MAC1 ==
  in0 : Inport  OutDataTypeStr=fixdt(1, 18, 16)  PortDimensions=[9 1]  SampleTime=1e-08
  in1 : Inport  Port=2  OutDataTypeStr=fixdt(1, 25, 12)  PortDimensions=[9]  SampleTime=1e-08
  globalSchedule : EnablePort  OutDataTypeStr=boolean
  PipelineRegister : Delay  DelayLength=double(8)  InitialCondition=0
  t : hdlsllib/HDL Operations/Multiply-Accumulate  opMode=Vector  initValueSetting=Dialog  initValue=0  initValueSetting2=Dialog  initValue2=0  initValueSetting3=Dialog  initValue3=0  num_samples=2  RndMeth2=Floor  RndMeth3=Floor  OutDataTypeStr=fixdt(1, 43, 28)  datatype2=Inherit: Inherit via back propagation  datatype3=Inherit: Inherit via back propagation  validOut=on  endInandOut=on  startOut=on  countOut=on  dim=-1  DoSatur=off  parallel=off
      settings: SourceProductBaseCode=SL
  out0 : Outport  OutDataTypeStr=fixdt(1, 43, 28)  SampleTime=1e-08  InitialOutput=0
  wires:
  PipelineRegister/1 -> out0/1
  in0/1 -> t/1
  in1/1 -> t/2
  t/1 -> PipelineRegister/1

== system gm_uz_pmsm_model_9ph/uz_pmsm_model_9ph/Transformation1/Transformation1_MAC2 ==
  in0 : Inport  OutDataTypeStr=fixdt(1, 18, 16)  PortDimensions=[9 1]  SampleTime=1e-08
  in1 : Inport  Port=2  OutDataTypeStr=fixdt(1, 25, 12)  PortDimensions=[9]  SampleTime=1e-08
  globalSchedule : EnablePort  OutDataTypeStr=boolean
  PipelineRegister : Delay  DelayLength=double(8)  InitialCondition=0
  t : hdlsllib/HDL Operations/Multiply-Accumulate  opMode=Vector  initValueSetting=Dialog  initValue=0  initValueSetting2=Dialog  initValue2=0  initValueSetting3=Dialog  initValue3=0  num_samples=2  RndMeth2=Floor  RndMeth3=Floor  OutDataTypeStr=fixdt(1, 43, 28)  datatype2=Inherit: Inherit via back propagation  datatype3=Inherit: Inherit via back propagation  validOut=on  endInandOut=on  startOut=on  countOut=on  dim=-1  DoSatur=off  parallel=off
      settings: SourceProductBaseCode=SL
  out0 : Outport  OutDataTypeStr=fixdt(1, 43, 28)  SampleTime=1e-08  InitialOutput=0
  wires:
  PipelineRegister/1 -> out0/1
  in0/1 -> t/1
  in1/1 -> t/2
  t/1 -> PipelineRegister/1

== system gm_uz_pmsm_model_9ph/uz_pmsm_model_9ph/Transformation1/Transformation1_MAC3 ==
  in0 : Inport  OutDataTypeStr=fixdt(1, 18, 16)  PortDimensions=[9 1]  SampleTime=1e-08
  in1 : Inport  Port=2  OutDataTypeStr=fixdt(1, 25, 12)  PortDimensions=[9]  SampleTime=1e-08
  globalSchedule : EnablePort  OutDataTypeStr=boolean
  PipelineRegister : Delay  DelayLength=double(8)  InitialCondition=0
  t : hdlsllib/HDL Operations/Multiply-Accumulate  opMode=Vector  initValueSetting=Dialog  initValue=0  initValueSetting2=Dialog  initValue2=0  initValueSetting3=Dialog  initValue3=0  num_samples=2  RndMeth2=Floor  RndMeth3=Floor  OutDataTypeStr=fixdt(1, 43, 28)  datatype2=Inherit: Inherit via back propagation  datatype3=Inherit: Inherit via back propagation  validOut=on  endInandOut=on  startOut=on  countOut=on  dim=-1  DoSatur=off  parallel=off
      settings: SourceProductBaseCode=SL
  out0 : Outport  OutDataTypeStr=fixdt(1, 43, 28)  SampleTime=1e-08  InitialOutput=0
  wires:
  PipelineRegister/1 -> out0/1
  in0/1 -> t/1
  in1/1 -> t/2
  t/1 -> PipelineRegister/1

== system gm_uz_pmsm_model_9ph/uz_pmsm_model_9ph/Transformation1/Transformation1_MAC4 ==
  in0 : Inport  OutDataTypeStr=fixdt(1, 18, 16)  PortDimensions=[9 1]  SampleTime=1e-08
  in1 : Inport  Port=2  OutDataTypeStr=fixdt(1, 25, 12)  PortDimensions=[9]  SampleTime=1e-08
  globalSchedule : EnablePort  OutDataTypeStr=boolean
  PipelineRegister : Delay  DelayLength=double(8)  InitialCondition=0
  t : hdlsllib/HDL Operations/Multiply-Accumulate  opMode=Vector  initValueSetting=Dialog  initValue=0  initValueSetting2=Dialog  initValue2=0  initValueSetting3=Dialog  initValue3=0  num_samples=2  RndMeth2=Floor  RndMeth3=Floor  OutDataTypeStr=fixdt(1, 43, 28)  datatype2=Inherit: Inherit via back propagation  datatype3=Inherit: Inherit via back propagation  validOut=on  endInandOut=on  startOut=on  countOut=on  dim=-1  DoSatur=off  parallel=off
      settings: SourceProductBaseCode=SL
  out0 : Outport  OutDataTypeStr=fixdt(1, 43, 28)  SampleTime=1e-08  InitialOutput=0
  wires:
  PipelineRegister/1 -> out0/1
  in0/1 -> t/1
  in1/1 -> t/2
  t/1 -> PipelineRegister/1

== system gm_uz_pmsm_model_9ph/uz_pmsm_model_9ph/Transformation1/Transformation1_MAC5 ==
  in0 : Inport  OutDataTypeStr=fixdt(1, 18, 16)  PortDimensions=[9 1]  SampleTime=1e-08
  in1 : Inport  Port=2  OutDataTypeStr=fixdt(1, 25, 12)  PortDimensions=[9]  SampleTime=1e-08
  globalSchedule : EnablePort  OutDataTypeStr=boolean
  PipelineRegister : Delay  DelayLength=double(8)  InitialCondition=0
  t : hdlsllib/HDL Operations/Multiply-Accumulate  opMode=Vector  initValueSetting=Dialog  initValue=0  initValueSetting2=Dialog  initValue2=0  initValueSetting3=Dialog  initValue3=0  num_samples=2  RndMeth2=Floor  RndMeth3=Floor  OutDataTypeStr=fixdt(1, 43, 28)  datatype2=Inherit: Inherit via back propagation  datatype3=Inherit: Inherit via back propagation  validOut=on  endInandOut=on  startOut=on  countOut=on  dim=-1  DoSatur=off  parallel=off
      settings: SourceProductBaseCode=SL
  out0 : Outport  OutDataTypeStr=fixdt(1, 43, 28)  SampleTime=1e-08  InitialOutput=0
  wires:
  PipelineRegister/1 -> out0/1
  in0/1 -> t/1
  in1/1 -> t/2
  t/1 -> PipelineRegister/1

== system gm_uz_pmsm_model_9ph/uz_pmsm_model_9ph/Transformation1/Transformation1_MAC6 ==
  in0 : Inport  OutDataTypeStr=fixdt(1, 18, 16)  PortDimensions=[9 1]  SampleTime=1e-08
  in1 : Inport  Port=2  OutDataTypeStr=fixdt(1, 25, 12)  PortDimensions=[9]  SampleTime=1e-08
  globalSchedule : EnablePort  OutDataTypeStr=boolean
  PipelineRegister : Delay  DelayLength=double(8)  InitialCondition=0
  t : hdlsllib/HDL Operations/Multiply-Accumulate  opMode=Vector  initValueSetting=Dialog  initValue=0  initValueSetting2=Dialog  initValue2=0  initValueSetting3=Dialog  initValue3=0  num_samples=2  RndMeth2=Floor  RndMeth3=Floor  OutDataTypeStr=fixdt(1, 43, 28)  datatype2=Inherit: Inherit via back propagation  datatype3=Inherit: Inherit via back propagation  validOut=on  endInandOut=on  startOut=on  countOut=on  dim=-1  DoSatur=off  parallel=off
      settings: SourceProductBaseCode=SL
  out0 : Outport  OutDataTypeStr=fixdt(1, 43, 28)  SampleTime=1e-08  InitialOutput=0
  wires:
  PipelineRegister/1 -> out0/1
  in0/1 -> t/1
  in1/1 -> t/2
  t/1 -> PipelineRegister/1

== system gm_uz_pmsm_model_9ph/uz_pmsm_model_9ph/Transformation1/Transformation1_MAC7 ==
  in0 : Inport  OutDataTypeStr=fixdt(1, 18, 16)  PortDimensions=[9 1]  SampleTime=1e-08
  in1 : Inport  Port=2  OutDataTypeStr=fixdt(1, 25, 12)  PortDimensions=[9]  SampleTime=1e-08
  globalSchedule : EnablePort  OutDataTypeStr=boolean
  PipelineRegister : Delay  DelayLength=double(8)  InitialCondition=0
  t : hdlsllib/HDL Operations/Multiply-Accumulate  opMode=Vector  initValueSetting=Dialog  initValue=0  initValueSetting2=Dialog  initValue2=0  initValueSetting3=Dialog  initValue3=0  num_samples=2  RndMeth2=Floor  RndMeth3=Floor  OutDataTypeStr=fixdt(1, 43, 28)  datatype2=Inherit: Inherit via back propagation  datatype3=Inherit: Inherit via back propagation  validOut=on  endInandOut=on  startOut=on  countOut=on  dim=-1  DoSatur=off  parallel=off
      settings: SourceProductBaseCode=SL
  out0 : Outport  OutDataTypeStr=fixdt(1, 43, 28)  SampleTime=1e-08  InitialOutput=0
  wires:
  PipelineRegister/1 -> out0/1
  in0/1 -> t/1
  in1/1 -> t/2
  t/1 -> PipelineRegister/1

== system gm_uz_pmsm_model_9ph/uz_pmsm_model_9ph/Transformation1/Transformation1_MAC8 ==
  in0 : Inport  OutDataTypeStr=fixdt(1, 18, 16)  PortDimensions=[9 1]  SampleTime=1e-08
  in1 : Inport  Port=2  OutDataTypeStr=fixdt(1, 25, 12)  PortDimensions=[9]  SampleTime=1e-08
  globalSchedule : EnablePort  OutDataTypeStr=boolean
  PipelineRegister : Delay  DelayLength=double(8)  InitialCondition=0
  t : hdlsllib/HDL Operations/Multiply-Accumulate  opMode=Vector  initValueSetting=Dialog  initValue=0  initValueSetting2=Dialog  initValue2=0  initValueSetting3=Dialog  initValue3=0  num_samples=2  RndMeth2=Floor  RndMeth3=Floor  OutDataTypeStr=fixdt(1, 43, 28)  datatype2=Inherit: Inherit via back propagation  datatype3=Inherit: Inherit via back propagation  validOut=on  endInandOut=on  startOut=on  countOut=on  dim=-1  DoSatur=off  parallel=off
      settings: SourceProductBaseCode=SL
  out0 : Outport  OutDataTypeStr=fixdt(1, 43, 28)  SampleTime=1e-08  InitialOutput=0
  wires:
  PipelineRegister/1 -> out0/1
  in0/1 -> t/1
  in1/1 -> t/2
  t/1 -> PipelineRegister/1

== system gm_uz_pmsm_model_9ph/uz_pmsm_model_9ph/Transformation1/t3 ==
  in0 : Inport
  ColVec1 : Selector  NumberOfDimensions=2  IndexOptions=Select all,Index vector (dialog)  Indices=1,1  OutputSizes=1,1
  ColVec2 : Selector  NumberOfDimensions=2  IndexOptions=Select all,Index vector (dialog)  Indices=1,2  OutputSizes=1,1
  ColVec3 : Selector  NumberOfDimensions=2  IndexOptions=Select all,Index vector (dialog)  Indices=1,3  OutputSizes=1,1
  ColVec4 : Selector  NumberOfDimensions=2  IndexOptions=Select all,Index vector (dialog)  Indices=1,4  OutputSizes=1,1
  ColVec5 : Selector  NumberOfDimensions=2  IndexOptions=Select all,Index vector (dialog)  Indices=1,5  OutputSizes=1,1
  ColVec6 : Selector  NumberOfDimensions=2  IndexOptions=Select all,Index vector (dialog)  Indices=1,6  OutputSizes=1,1
  ColVec7 : Selector  NumberOfDimensions=2  IndexOptions=Select all,Index vector (dialog)  Indices=1,7  OutputSizes=1,1
  ColVec8 : Selector  NumberOfDimensions=2  IndexOptions=Select all,Index vector (dialog)  Indices=1,8  OutputSizes=1,1
  ColVec9 : Selector  NumberOfDimensions=2  IndexOptions=Select all,Index vector (dialog)  Indices=1,9  OutputSizes=1,1
  out0 : Outport
  out1 : Outport  Port=2
  out2 : Outport  Port=3
  out3 : Outport  Port=4
  out4 : Outport  Port=5
  out5 : Outport  Port=6
  out6 : Outport  Port=7
  out7 : Outport  Port=8
  out8 : Outport  Port=9
  wires:
  in0/1 -> ColVec1/1, ColVec2/1, ColVec3/1, ColVec4/1, ColVec5/1, ColVec6/1, ColVec7/1, ColVec8/1, ColVec9/1
  ColVec1/1 -> out0/1
  ColVec2/1 -> out1/1
  ColVec3/1 -> out2/1
  ColVec4/1 -> out3/1
  ColVec5/1 -> out4/1
  ColVec6/1 -> out5/1
  ColVec7/1 -> out6/1
  ColVec8/1 -> out7/1
  ColVec9/1 -> out8/1

== system gm_uz_pmsm_model_9ph/uz_pmsm_model_9ph/Wrapped State DTI/Compare To Constant1_relop ==
  In1 : Inport
  In2 : Inport  Port=2
  Compare To Constant1_relop : RelationalOperator  Operator=<  OutDataTypeStr=boolean  SampleTime=1e-08  RndMeth=Nearest  InputSameDT=on
  Compare To Constant1_relop_pd1 : Delay  DelayLength=1
  Out1 : Outport
  wires:
  In1/1 -> Compare To Constant1_relop/1
  In2/1 -> Compare To Constant1_relop/2
  Compare To Constant1_relop/1 -> Compare To Constant1_relop_pd1/1
  Compare To Constant1_relop_pd1/1 -> Out1/1

== system gm_uz_pmsm_model_9ph/uz_pmsm_model_9ph/Wrapped State DTI/Compare To Constant_relop ==
  In1 : Inport
  In2 : Inport  Port=2
  Compare To Constant_relop : RelationalOperator  OutDataTypeStr=boolean  SampleTime=1e-08  RndMeth=Nearest  InputSameDT=on
  Compare To Constant_relop_pd1 : Delay  DelayLength=1
  Out1 : Outport
  wires:
  In1/1 -> Compare To Constant_relop/1
  In2/1 -> Compare To Constant_relop/2
  Compare To Constant_relop/1 -> Compare To Constant_relop_pd1/1
  Compare To Constant_relop_pd1/1 -> Out1/1

== system gm_uz_pmsm_model_9ph/uz_pmsm_model_9ph/Wrapped State DTI/Gain ==
  In1 : Inport
  In2 : Inport  Port=2
  Gain : Product  Inputs=**  OutDataTypeStr=single  SampleTime=1e-08
  Gain_pd1 : Delay  DelayLength=6
  Out1 : Outport
  wires:
  In1/1 -> Gain/1
  In2/1 -> Gain/2
  Gain/1 -> Gain_pd1/1
  Gain_pd1/1 -> Out1/1

== system gm_uz_pmsm_model_9ph/uz_pmsm_model_9ph/Wrapped State DTI/Product ==
  In1 : Inport
  In2 : Inport  Port=2
  Product : Product  Inputs=**  OutDataTypeStr=single  SampleTime=1e-08
  Product_pd1 : Delay  DelayLength=6
  Out1 : Outport
  wires:
  In1/1 -> Product/1
  In2/1 -> Product/2
  Product/1 -> Product_pd1/1
  Product_pd1/1 -> Out1/1

== system gm_uz_pmsm_model_9ph/uz_pmsm_model_9ph/Wrapped State DTI/Sum ==
  In1 : Inport
  In2 : Inport  Port=2
  Sum : Sum  OutDataTypeStr=single  SampleTime=1e-08
  Sum_pd1 : Delay  DelayLength=6
  Out1 : Outport
  wires:
  In1/1 -> Sum/1
  In2/1 -> Sum/2
  Sum/1 -> Sum_pd1/1
  Sum_pd1/1 -> Out1/1

== system gm_uz_pmsm_model_9ph/uz_pmsm_model_9ph/Wrapped State DTI/Sum1 ==
  In1 : Inport
  In2 : Inport  Port=2
  Sum1 : Sum  Inputs=+-  OutDataTypeStr=single  SampleTime=1e-08
  Sum1_pd1 : Delay  DelayLength=6
  Out1 : Outport
  wires:
  In1/1 -> Sum1/1
  In2/1 -> Sum1/2
  Sum1/1 -> Sum1_pd1/1
  Sum1_pd1/1 -> Out1/1

== system gm_uz_pmsm_model_9ph/uz_pmsm_model_9ph/Wrapped State DTI/Sum2 ==
  In1 : Inport
  In2 : Inport  Port=2
  Sum2 : Sum  OutDataTypeStr=single  SampleTime=1e-08
  Sum2_pd1 : Delay  DelayLength=6
  Out1 : Outport
  wires:
  In1/1 -> Sum2/1
  In2/1 -> Sum2/2
  Sum2/1 -> Sum2_pd1/1
  Sum2_pd1/1 -> Out1/1

== system gm_uz_pmsm_model_9ph/uz_pmsm_model_9ph/Line-Line to Phase voltage/abc   to   alpha_beta_0/Gain2 ==
  In1 : Inport
  In2 : Inport  Port=2
  Gain2 : Product  Inputs=**  OutDataTypeStr=single  SaturateOnIntegerOverflow=on  SampleTime=1e-08
  Gain2_pd1 : Delay  DelayLength=6
  Out1 : Outport
  wires:
  In1/1 -> Gain2/1
  In2/1 -> Gain2/2
  Gain2/1 -> Gain2_pd1/1
  Gain2_pd1/1 -> Out1/1

== system gm_uz_pmsm_model_9ph/uz_pmsm_model_9ph/Line-Line to Phase voltage/abc   to   alpha_beta_0/MMul_add_01 ==
  In1 : Inport
  In2 : Inport  Port=2
  MMul_add_01 : Sum  OutDataTypeStr=single  SampleTime=1e-08
  MMul_add_01_pd1 : Delay  DelayLength=6
  Out1 : Outport
  wires:
  In1/1 -> MMul_add_01/1
  In2/1 -> MMul_add_01/2
  MMul_add_01/1 -> MMul_add_01_pd1/1
  MMul_add_01_pd1/1 -> Out1/1
